simulink model "pwm2"  (Simulink 8.3)
settings: Solver=ode45  StartTime=0.0  StopTime=5  RelTol=1e-3
undefined symbols (not defined in the file): m
libraries: powerlib x16, powerlib_meascontrol x1
settings Model: Creator=lenovo  LastModifiedBy=lenovo
settings DataIOCC: SignalLoggingSaveFormat=Dataset
settings DebuggingCC: UnderspecifiedInitializationDetection=Simplified  UnconnectedLineMsg=none  StateNameClashWarn=none
settings GRTTargetCC: CombineOutputUpdateFcns=on  GRTInterface=off

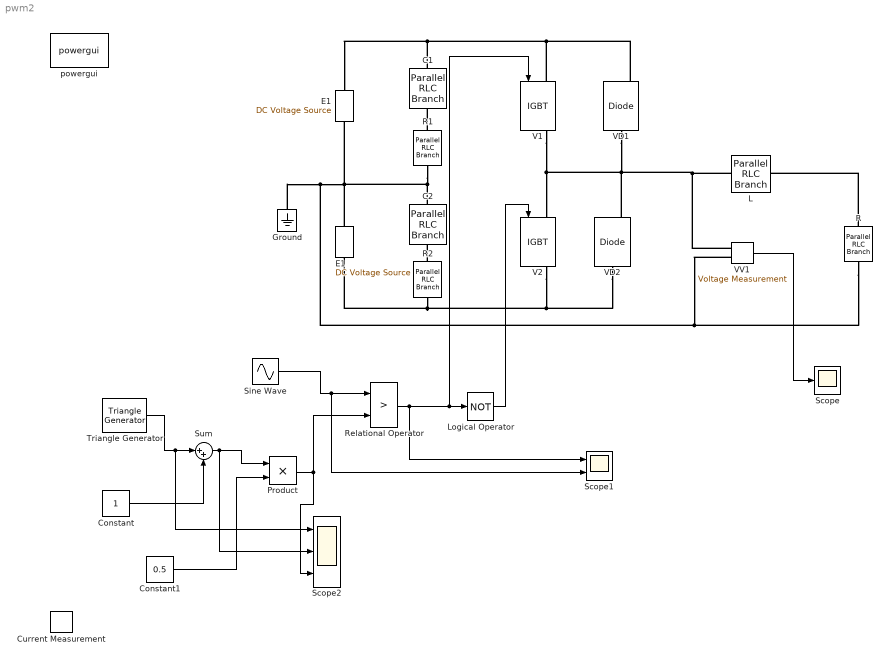
== system pwm2 ==
  C1 : powerlib/Elements/Parallel RLC Branch  LConnTagsString=a  RConnTagsString=__new0  BranchType=C  Resistance=inf  Inductance=1e-3  SetiL0=off  InitialCurrent=0  Capacitance=1e-3  Setx0=off  InitialVoltage=0  Measurements=None
  C2 : powerlib/Elements/Parallel RLC Branch  LConnTagsString=a  RConnTagsString=__new0  BranchType=C  Resistance=inf  Inductance=1e-3  SetiL0=off  InitialCurrent=0  Capacitance=1e-3  Setx0=off  InitialVoltage=0  Measurements=None
  Constant : Constant
  Constant1 : Constant  Value=0.5
  Current Measurement : powerlib/Measurements/Current Measurement  PhasorSimulation=off  OutputType=Complex  PSBequivalent=0
  E1 : powerlib/Electrical Sources/DC Voltage Source  Amplitude=10  Measurements=None
  "E1 " : powerlib/Electrical Sources/DC Voltage Source  Amplitude=10  Measurements=None
  Ground : powerlib/Elements/Ground  LConnTagsString=a
  L : powerlib/Elements/Parallel RLC Branch  LConnTagsString=a  RConnTagsString=__new0  BranchType=L  Resistance=inf  Inductance=1e-3  SetiL0=off  InitialCurrent=0  Capacitance=inf  Setx0=off  InitialVoltage=0  Measurements=None
  Logical Operator : Logic  Operator=NOT  AllPortsSameDT=off  OutDataTypeStr=boolean
  Product : Product
  R : powerlib/Elements/Parallel RLC Branch  LConnTagsString=a  RConnTagsString=__new0  BranchType=R  Resistance=400  Inductance=1e-3  SetiL0=off  InitialCurrent=0  Capacitance=inf  Setx0=off  InitialVoltage=0  Measurements=None
  R1 : powerlib/Elements/Parallel RLC Branch  LConnTagsString=a  RConnTagsString=__new0  BranchType=R  Resistance=1e-8  Inductance=1e-3  SetiL0=off  InitialCurrent=0  Capacitance=inf  Setx0=off  InitialVoltage=0  Measurements=None
  R2 : powerlib/Elements/Parallel RLC Branch  LConnTagsString=a  RConnTagsString=__new0  BranchType=R  Resistance=1e-8  Inductance=1e-3  SetiL0=off  InitialCurrent=0  Capacitance=inf  Setx0=off  InitialVoltage=0  Measurements=None
  Relational Operator : RelationalOperator  Operator=>  OutDataTypeStr=boolean
  Scope : Scope
      settings: YMax=20
  Scope1 : Scope  NumInputPorts=2
      settings: YMin=0~0  YMax=1.5~1  MaxDataPoints=500000
  Scope2 : Scope  NumInputPorts=3
      settings: YMin=-1~-2~0  YMax=2~2~1  SaveName=ScopeData2  MaxDataPoints=500000
  Sine Wave : Sin  Amplitude=0.5*m  Bias=0.5  Frequency=2*pi*50  Phase=0.25*pi  SampleTime=0
  Sum : Sum  Inputs=|++
  Triangle Generator : powerlib_meascontrol/Pulse & Signal Generators/Triangle Generator  Freq=1e3  Phase=90  Ts=0
  V1 : powerlib/Power Electronics/IGBT  Ron=1e-6  Lon=0  Vf=0  Tf=1e-6  Tt=2e-6  IC=0  Rs=1e5  Cs=inf  Measurements=on
  V2 : powerlib/Power Electronics/IGBT  Ron=1e-6  Lon=0  Vf=0  Tf=1e-6  Tt=2e-6  IC=0  Rs=1e5  Cs=inf  Measurements=on
  VD1 : powerlib/Power Electronics/Diode  Ron=1e-6  Lon=0  Vf=0.8  IC=0  UseSnubber=off  Rs=inf  Cs=250e-9  Measurements=on
  VD2 : powerlib/Power Electronics/Diode  Ron=1e-6  Lon=0  Vf=0.8  IC=0  UseSnubber=off  Rs=inf  Cs=250e-9  Measurements=on
  VV1 : powerlib/Measurements/Voltage Measurement  PhasorSimulation=off  OutputType=Complex  PSBequivalent=0
  powergui : powerlib/powergui  Priority=1  SimulationMode=Discrete  SolverType=Tustin  SampleTime=1e-6  frequency=60  SPID=off  DisableSnubberDevices=on  DisableRonSwitches=on  DisableVfSwitches=on  SwTol=0  Interpol=off  DisplayEquations=on  Ts=0  methode=off  frequencyindice=0  Pbase=100e6  ErrMax=1e-4  Iterations=50  UnitsV=V  UnitsW=W  FunctionMessages=off  echomessages=off  HookPort=off  EnableUseOfTLC=off  x0status=blocks  RestoreLinks=warning  ResistiveCurrentMeasurement=off  Frange=[0:2:500]  Ylog=off  Xlog=on  ShowGrid=off  save=off  variable=ZData  structure=0  ZoomFFT=off  StartTime=0.0  cycles=1  DisplayStyle=1  fundamental=60  FreqAxis=off  MaxFrequency=1000  frequencyindicesteady=1  RmsSteady=1  display=off
  wires:
  Sine Wave/1 -> Scope1/2, Relational Operator/1
  VV1/1 -> Scope/1
  Relational Operator/1 -> Scope1/1, V1/1, Logical Operator/1
  Logical Operator/1 -> V2/1
  Triangle Generator/1 -> Scope2/1, Sum/1
  Constant/1 -> Sum/2
  Sum/1 -> Scope2/2, Product/1
  Constant1/1 -> Product/2
  Product/1 -> Relational Operator/2, Scope2/3
  connections:
  "E1 "/RConn1 -- C2/LConn1 -- R1/RConn1 -- VV1/LConn2 -- R/RConn1 -- Ground/LConn1 -- E1/LConn1
  V1/LConn1 -- VD1/RConn1 -- C1/LConn1 -- E1/RConn1
  V1/RConn1 -- VV1/LConn1 -- L/LConn1 -- VD1/LConn1 -- VD2/RConn1 -- V2/LConn1
  V2/RConn1 -- VD2/LConn1 -- R2/RConn1 -- "E1 "/LConn1
  R/LConn1 -- L/RConn1
  R1/LConn1 -- C1/RConn1
  R2/LConn1 -- C2/RConn1
